simulink model "UdpRealTime"  (R2017b)
settings: Solver=FixedStepDiscrete  StartTime=0.0  StopTime=inf  FixedStep=0.0005  RelTol=1e-3  EnableMultiTasking=on
undefined symbols (not defined in the file or in its folder): BusModule, CassieModule
libraries: xpcrtudplib x2, CassieLibrary x1, slrtlib x1
settings Model: xpc_rtwmakecfg_data=_xpcethercatlib_  Creator=Patrick  LastModifiedBy=PatrickClary
settings DataIOCC: SaveFormat=Array  SaveOutput=off  SignalLogging=off  DSMLogging=off  SaveTime=off
settings OptimizationCC: DefaultParameterBehavior=Inlined  InlineInvariantSignals=on  LifeSpan=inf  SimCompilerOptimization=on  AccelVerboseBuild=on
settings DebuggingCC: AllowSymbolicDim=off
settings HardwareCC: ProdBitPerPointer=32  ProdBitPerSizeT=32  ProdBitPerPtrDiffT=32  ProdLargestAtomicFloat=None  ProdWordSize=32  ProdLongLongMode=on  ProdHWDeviceType=Generic->32-bit x86 compatible
settings ModelReferenceCC: ModelReferenceNumInstancesAllowed=Zero
settings SFSimCC: SFSimEcho=off
settings RTWCC: SystemTargetFile=slrt.tlc  TLCOptions=-axPCMaxOverloads=1000000000 -axPCMaxOverloadLen=1000000000  TemplateMakefile=slrt_default_tmf  Description=Simulink Real-Time  CodeExecutionProfiling=on  RTWCompilerOptimization=on
settings CodeAppCC: GenerateComments=off  MaxIdLength=128  SimulinkBlockComments=off

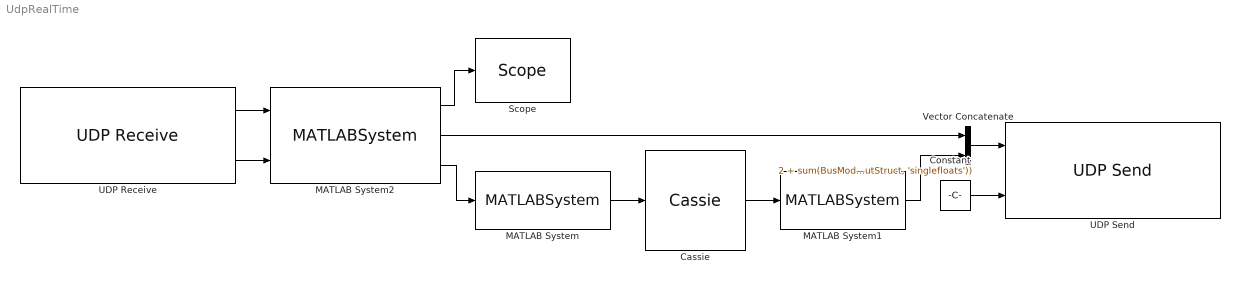
== system UdpRealTime ==
  Cassie : CassieLibrary/RealTime/Cassie  SystemSampleTime=-1
  Constant : Constant  Value=2 + sum(BusModule.getPackingInfo(CassieModule.getOutStruct, 'singlefloats'))
  MATLAB System : MATLABSystem  System=BytesToCassieUserInBus  SimulateUsing=Code generation
      mask Type: BytesToCassieUserInBus
      mask Display: disp('BytesToCassieUserInBus');
  MATLAB System1 : MATLABSystem  System=CassieOutBusToBytes  SimulateUsing=Code generation
      mask Type: CassieOutBusToBytes
      mask Display: disp('CassieOutBusToBytes');
  MATLAB System2 : MATLABSystem  System=ProcessUdpPacket  heartbeatInterval=0.01  dataLength=sum(BusModule.getPackingInfo(CassieModule.getUserInStruct, 'singlefloats'))  SimulateUsing=Code generation
      mask Type: ProcessUdpPacket
      mask Display:
      | disp('ProcessUdpPacket');
      | port_label('input',1,'UDP Data');
      | port_label('input',2,'Length');
      | port_label('output',1,'Log');
      | port_label('output',2,'Header');
      | port_label('output',3,'Data');
  "Scope " : slrtlib/Displays and Logging/Scope   scopeno=2  scopetype=File  autostart=on  viewmode=Graphical redraw  formatstr='%15.6f'  grid=on  ylimits=[0,0]  nosamples=250  noprepostsamples=0  interleave=1  triggermode=FreeRun  triggersignal=1  trigsignalfromport=off  triggerlevel=0.0  triggerslope=Either  triggerscope=1  triggersample=0  filename=udp.dat  mode=Commit  writesize=4096  autorestart=on  dynamicfilemode=off  maxwritefilesize=2048*1024^2 - 4096
  UDP Receive : xpcrtudplib/UDP Receive  ipAddressVal=Use host-target connection  localPort=25000  rcvWidth=2 + sum(BusModule.getPackingInfo(CassieModule.getUserInStruct, 'singlefloats'))  rcvFmAny=off  fmAddress=10.10.10.100  maxUDPQueue=8  sampleTime=-1
      settings: SourceProductName=Simulink Real-Time
  UDP Send : xpcrtudplib/UDP Send  ipAddressVal=Use host-target connection  localPort=25000  toAddress=10.10.10.100  toPort=25001  sampleTime=-1
      settings: SourceProductName=Simulink Real-Time  SourceProductBaseCode=XP
  Vector Concatenate : Concatenate
  wires:
  Cassie/1 -> MATLAB System1/1
  MATLAB System/1 -> Cassie/1
  Constant/1 -> UDP Send/2
  MATLAB System2/3 -> MATLAB System/1
  UDP Receive/2 -> MATLAB System2/2
  MATLAB System1/1 -> Vector Concatenate/2
  Vector Concatenate/1 -> UDP Send/1
  UDP Receive/1 -> MATLAB System2/1
  MATLAB System2/2 -> Vector Concatenate/1
  MATLAB System2/1 -> "Scope "/1
